simulink library "astrobee_linear_pos_ctl_lib"  (R2015b)
settings: Solver=VariableStepAuto  StartTime=0.0  StopTime=10.0  RelTol=1e-3
undefined symbols (not defined in the file): tun_abp_veh_mass, tun_ctl_pos_Ti, tun_ctl_pos_Tp, tun_ctl_vel_kd
settings Model: Creator=jfusco1  LastModifiedBy=jfusco1

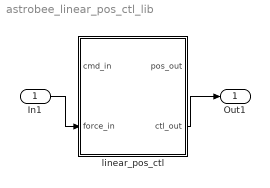
== system astrobee_linear_pos_ctl_lib ==
  In1 : Inport  PortDimensions=3
  linear_pos_ctl : Subsystem
  Out1 : Outport
  wires:
  In1/1 -> linear_pos_ctl/2(force_in)
  linear_pos_ctl/2(ctl_out) -> Out1/1

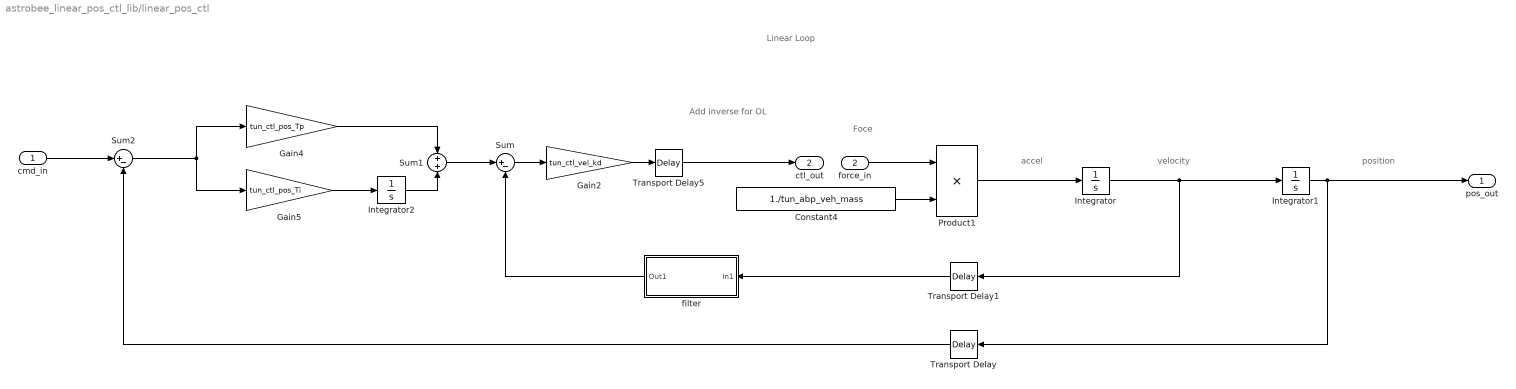
== system astrobee_linear_pos_ctl_lib/linear_pos_ctl ==
  note: Foce
  note: accel
  note: velocity
  note: position
  note: Linear Loop
  note: Add inverse for OL
  cmd_in : Inport
  force_in : Inport  Port=2  PortDimensions=3
  Constant4 : Constant  Value=1./tun_abp_veh_mass
  Gain2 : Gain  Gain=tun_ctl_vel_kd
  Gain4 : Gain  Gain=tun_ctl_pos_Tp
  Gain5 : Gain  Gain=tun_ctl_pos_Ti
  Integrator : Integrator
  Integrator1 : Integrator
  Integrator2 : Integrator
  Product1 : Product
  Sum : Sum  Inputs=|+-
  Sum1 : Sum  Inputs=+|+
  Sum2 : Sum  Inputs=|+-
  Transport Delay : TransportDelay  DelayTime=1/62.5  PadeOrder=5
  Transport Delay1 : TransportDelay  DelayTime=1/62.5  PadeOrder=5
  Transport Delay5 : TransportDelay  DelayTime=1/62.5  PadeOrder=5
  filter : Subsystem  TreatAsAtomicUnit=on
  pos_out : Outport
  ctl_out : Outport  Port=2
  wires:
  Constant4/1 -> Product1/2
  Sum/1 -> Gain2/1
  Product1/1 -> Integrator/1
  Integrator/1 -> Transport Delay1/1, Integrator1/1
  Integrator1/1 -> pos_out/1, Transport Delay/1
  Gain5/1 -> Integrator2/1
  Integrator2/1 -> Sum1/2
  Gain4/1 -> Sum1/1
  Sum1/1 -> Sum/1
  Sum2/1 -> Gain5/1, Gain4/1
  Transport Delay/1 -> Sum2/2
  cmd_in/1 -> Sum2/1
  Gain2/1 -> Transport Delay5/1
  Transport Delay5/1 -> ctl_out/1
  force_in/1 -> Product1/1
  Transport Delay1/1 -> filter/1(In1)
  filter/1(Out1) -> Sum/2

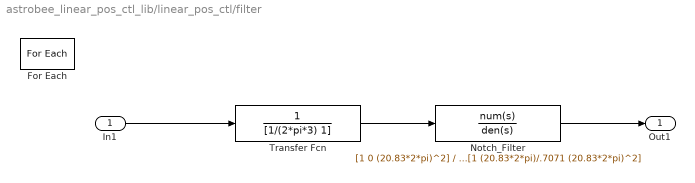
== system astrobee_linear_pos_ctl_lib/linear_pos_ctl/filter ==
  In1 : Inport  Partition=on  PartitionDimension=1  PartitionWidth=1
  For Each : ForEach  DisableCoverage=on  IndexMode=One-based
  Notch_Filter : TransferFcn  Numerator=[1 0 (20.83*2*pi)^2]  Denominator=[1 (20.83*2*pi)/.7071 (20.83*2*pi)^2]
  Transfer Fcn : TransferFcn  Denominator=[1/(2*pi*3) 1]
  Out1 : Outport  ConcatenationDimension=1
  wires:
  In1/1 -> Transfer Fcn/1
  Transfer Fcn/1 -> Notch_Filter/1
  Notch_Filter/1 -> Out1/1
